simulink model "simulation"  (R2018b)
settings: Solver=ode45  StartTime=0.0  StopTime=inf  MaxStep=0.01  RelTol=1e-3
values from neighbouring files (symbols this model uses):
  A_ref = pi*r^2    (= 0.0188691908756)    [inputsSimulink.m]    (also in stability.m = Geometria(11))
  Cd_lateral1 = Cd_lateral1*A_lateral1/A_ref    (= 119.241996905)    [inputsSimulink.m]
  Cd_lateral2 = Cd_lateral2*A_lateral2/A_ref    (= 238.483993811)    [inputsSimulink.m]
  Cd_paraquedas1 = Cd_paraquedas1*A_paraquedas1/A_ref    (= 24.6433460271)    [inputsSimulink.m]
  Cd_paraquedas2 = Cd_paraquedas2*A_paraquedas2/A_ref    (= 483.857525221)    [inputsSimulink.m]
  Cn = Cn_SB    [inputsSimulink.m]    (also in stability.m = CN_bosters + CN)
  dist_guia = 12    [inputsSimulink.m]
  Empuxo_boster = 4*curvas(:,2)    [inputsSimulink.m]
  g0 = 9.82    [inputsSimulink.m]
  h0 = 1200    [inputsSimulink.m]
  L_coifa = 0.5    [inputsSimulink.m]    (also in stability.m = Geometria(3))
  L_corpo = 2    [inputsSimulink.m]
  Massa_foguete = 1    [inputsSimulink.m]
  Massa_motor_solido = [3.5 1]    [inputsSimulink.m]
  ME = (Cp - CG)/(2*r)    [inputsSimulink.m]
  phi = 0    [inputsSimulink.m]
  r = 0.155/2    (= 0.0775)    [inputsSimulink.m]    (also in stability.m = Geometria(1))
  RE = 6371000    [inputsSimulink.m]
  tempo_abertura1 = 5    [inputsSimulink.m]
  tempo_abertura2 = 7    [inputsSimulink.m]
  tempo_boster = curvas(:,1)    [inputsSimulink.m]
  tempo_motor_solido = [0 tempo_queima_bosters]    [inputsSimulink.m]
  tempo_queima_bosters = max(tempo_boster)    [inputsSimulink.m]
  theta = 0    [inputsSimulink.m]
  Vento_eixo_x = 1    [inputsSimulink.m]
  Vento_eixo_y = 0    [inputsSimulink.m]
libraries: vrlib x3, aerolibatmos2 x1
settings Model: Creator=root  LastModifiedBy=root

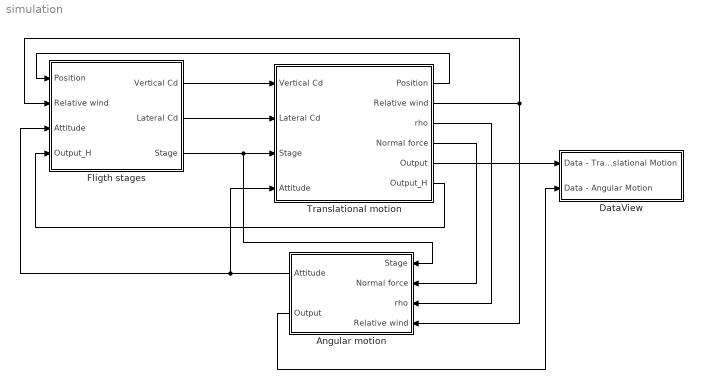
== system simulation ==
  Angular motion : Subsystem
  DataView : Subsystem
  Fligth stages : Subsystem
  Translational motion : Subsystem
  wires:
  Fligth stages/1(Vertical Cd) -> Translational motion/1(Vertical Cd)
  Translational motion/4(Normal force) -> Angular motion/2(Normal force)
  Translational motion/6(Output_H) -> Fligth stages/4(Output_H)
  Translational motion/3(rho) -> Angular motion/3(rho)
  Fligth stages/2(Lateral Cd) -> Translational motion/2(Lateral Cd)
  Fligth stages/3(Stage) -> Angular motion/1(Stage), Translational motion/3(Stage)
  Translational motion/1(Position) -> Fligth stages/1(Position)
  Angular motion/1(Attitude) -> Fligth stages/3(Attitude), Translational motion/4(Attitude)
  Translational motion/2(Relative wind) -> Fligth stages/2(Relative wind), Angular motion/4(Relative wind)
  Translational motion/5(Output) -> DataView/1(Data - Translational Motion)
  Angular motion/2(Output) -> DataView/2(Data - Angular Motion)

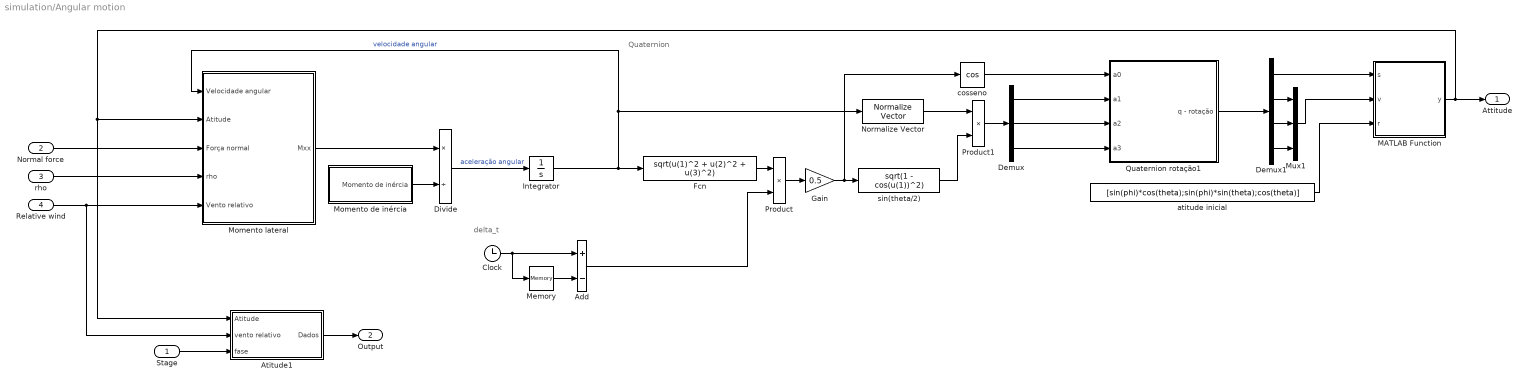
== system simulation/Angular motion ==
  note: Quaternion
  note: delta_t
  Stage : Inport
  Normal force : Inport  Port=2
  rho : Inport  Port=3
  Relative wind : Inport  Port=4
  Add : Sum  Inputs=+-
  Atitude1 : Subsystem
  Clock : Clock
  Demux : Demux  Outputs=3
  Demux1 : Demux
  Divide : Product  Inputs=*/
  Fcn : Fcn  Expr=sqrt(u(1)^2 + u(2)^2 + u(3)^2)
  Gain : Gain  Gain=0.5
  Integrator : Integrator  InitialCondition=[0;0;0]
  MATLAB Function : MATLAB Function  TreatAsAtomicUnit=on
  Memory : Memory
  Momento de inércia : Subsystem
  Momento lateral : Subsystem
  Mux1 : Mux  Inputs=3
  Normalize Vector : vrlib/Utilities/Normalize Vector  maxzero=0
      settings: SourceProductName=Simulink 3D Animation  SourceProductBaseCode=VR
  Product : Product
  Product1 : Product
  Quaternion rotação1 : Subsystem
  atitude inicial : Constant  Value=[sin(phi)*cos(theta);sin(phi)*sin(theta);cos(theta)]
  cosseno : Trigonometry  Operator=cos
  sin(theta/2) : Fcn  Expr=sqrt(1 - cos(u(1))^2)
  Attitude : Outport
  Output : Outport  Port=2
  wires:
  Normal force/1 -> Momento lateral/3(Força normal)
  rho/1 -> Momento lateral/4(rho)
  Relative wind/1 -> Momento lateral/5(Vento relativo), Atitude1/2(vento relativo)
  Momento lateral/1(Mxx) -> Divide/1
  Momento de inércia/1(Momento de inércia) -> Divide/2
  Divide/1 -> Integrator/1  "aceleração angular"
  Clock/1 -> Memory/1, Add/1
  Memory/1 -> Add/2
  Integrator/1 -> Normalize Vector/1, Momento lateral/1(Velocidade angular), Fcn/1  "velocidade angular"
  Add/1 -> Product/2
  Product/1 -> Gain/1
  Gain/1 -> cosseno/1, sin(theta/2)/1
  sin(theta/2)/1 -> Product1/2
  Product1/1 -> Demux/1
  cosseno/1 -> Quaternion rotação1/1(a0)
  atitude inicial/1 -> MATLAB Function/3(r)
  MATLAB Function/1(y) -> Atitude1/1(Atitude), Momento lateral/2(Atitude), Attitude/1
  Fcn/1 -> Product/1
  Normalize Vector/1 -> Product1/1
  Demux/3 -> Quaternion rotação1/4(a3)
  Demux/2 -> Quaternion rotação1/3(a2)
  Demux/1 -> Quaternion rotação1/2(a1)
  Demux1/1 -> MATLAB Function/1(s)
  Demux1/4 -> Mux1/3
  Demux1/3 -> Mux1/2
  Demux1/2 -> Mux1/1
  Mux1/1 -> MATLAB Function/2(v)
  Quaternion rotação1/1(q - rotação) -> Demux1/1
  Stage/1 -> Atitude1/3(fase)
  Atitude1/1(Dados) -> Output/1

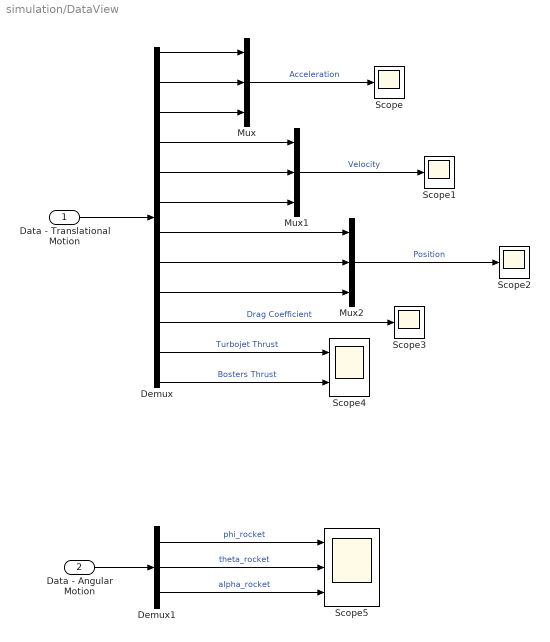
== system simulation/DataView ==
  Data - Translational Motion : Inport
  Data - Angular Motion : Inport  Port=2
  Demux : Demux  Outputs=12
  Demux1 : Demux  Outputs=3
  Mux : Mux  Inputs=3
  Mux1 : Mux  Inputs=3
  Mux2 : Mux  Inputs=3
  Scope{,1..3} (4 alike) : Scope
  Scope4 : Scope  NumInputPorts=2
  Scope5 : Scope  NumInputPorts=3
  wires:
  Data - Translational Motion/1 -> Demux/1
  Demux/1 -> Mux/1
  Demux/2 -> Mux/2
  Demux/3 -> Mux/3
  Demux/4 -> Mux1/1
  Demux/5 -> Mux1/2
  Demux/6 -> Mux1/3
  Demux/7 -> Mux2/1
  Demux/8 -> Mux2/2
  Demux/9 -> Mux2/3
  Mux/1 -> Scope/1  "Acceleration"
  Mux1/1 -> Scope1/1  "Velocity"
  Mux2/1 -> Scope2/1  "Position"
  Demux/10 -> Scope3/1  "Drag Coefficient"
  Demux/11 -> Scope4/1  "Turbojet Thrust"
  Demux/12 -> Scope4/2  "Bosters Thrust"
  Data - Angular Motion/1 -> Demux1/1
  Demux1/2 -> Scope5/2  "theta_rocket"
  Demux1/3 -> Scope5/3  "alpha_rocket"
  Demux1/1 -> Scope5/1  "phi_rocket"

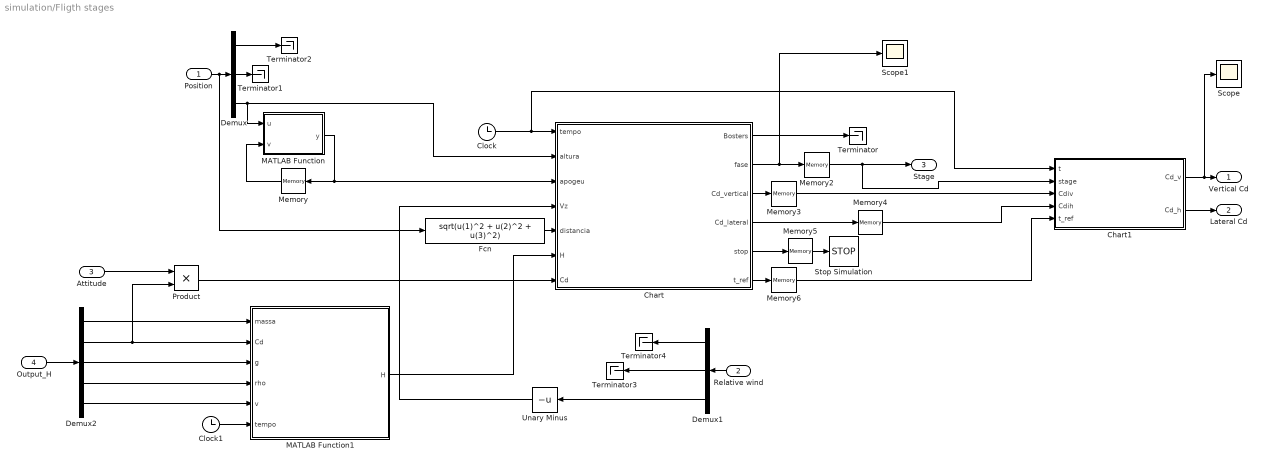
== system simulation/Fligth stages ==
  Position : Inport
  Relative wind : Inport  Port=2
  Attitude : Inport  Port=3
  Output_H : Inport  Port=4
  Chart : Stateflow chart  TreatAsAtomicUnit=on
  Chart1 : Stateflow chart  TreatAsAtomicUnit=on
  Clock : Clock
  Clock1 : Clock
  Demux : Demux  Outputs=3
  Demux1 : Demux  Outputs=3
  Demux2 : Demux  Outputs=5
  Fcn : Fcn  Expr=sqrt(u(1)^2 + u(2)^2 + u(3)^2)
  MATLAB Function : MATLAB Function  TreatAsAtomicUnit=on
  MATLAB Function1 : MATLAB Function  TreatAsAtomicUnit=on
  Memory{,2..6} (6 alike) : Memory
  Product : Product
  Scope : Scope
  Scope1 : Scope
  Stop Simulation : Stop
  Terminator{,1..4} (5 alike) : Terminator
  Unary Minus : UnaryMinus
  Vertical Cd : Outport
  Lateral Cd : Outport  Port=2
  Stage : Outport  Port=3
  wires:
  Demux/3 -> MATLAB Function/1(u), Chart/2(altura)
  Chart/2(fase) -> Scope1/1, Memory2/1
  Chart/3(Cd_vertical) -> Memory3/1
  Chart/4(Cd_lateral) -> Memory4/1
  Position/1 -> Fcn/1, Demux/1
  Demux/2 -> Terminator1/1
  Demux/1 -> Terminator2/1
  Chart/5(stop) -> Memory5/1
  Relative wind/1 -> Demux1/1
  Demux1/2 -> Terminator3/1
  Demux1/1 -> Terminator4/1
  Demux1/3 -> Unary Minus/1
  Unary Minus/1 -> Chart/4(Vz)
  Fcn/1 -> Chart/5(distancia)
  MATLAB Function/1(y) -> Chart/3(apogeu), Memory/1
  Memory/1 -> MATLAB Function/2(v)
  Output_H/1 -> Demux2/1
  Demux2/1 -> MATLAB Function1/1(massa)
  Demux2/2 -> Product/2, MATLAB Function1/2(Cd)
  Demux2/3 -> MATLAB Function1/3(g)
  Demux2/4 -> MATLAB Function1/4(rho)
  Demux2/5 -> MATLAB Function1/5(v)
  MATLAB Function1/1(H) -> Chart/6(H)
  Clock/1 -> Chart1/1(t), Chart/1(tempo)
  Chart/6(t_ref) -> Memory6/1
  Chart1/2(Cd_h) -> Lateral Cd/1
  Attitude/1 -> Product/1
  Product/1 -> Chart/7(Cd)
  Clock1/1 -> MATLAB Function1/6(tempo)
  Memory2/1 -> Stage/1, Chart1/2(stage)
  Memory3/1 -> Chart1/3(Cdiv)
  Memory4/1 -> Chart1/4(Cdih)
  Memory5/1 -> Stop Simulation/1
  Memory6/1 -> Chart1/5(t_ref)
  Chart1/1(Cd_v) -> Scope/1, Vertical Cd/1
  Chart/1(Bosters) -> Terminator/1

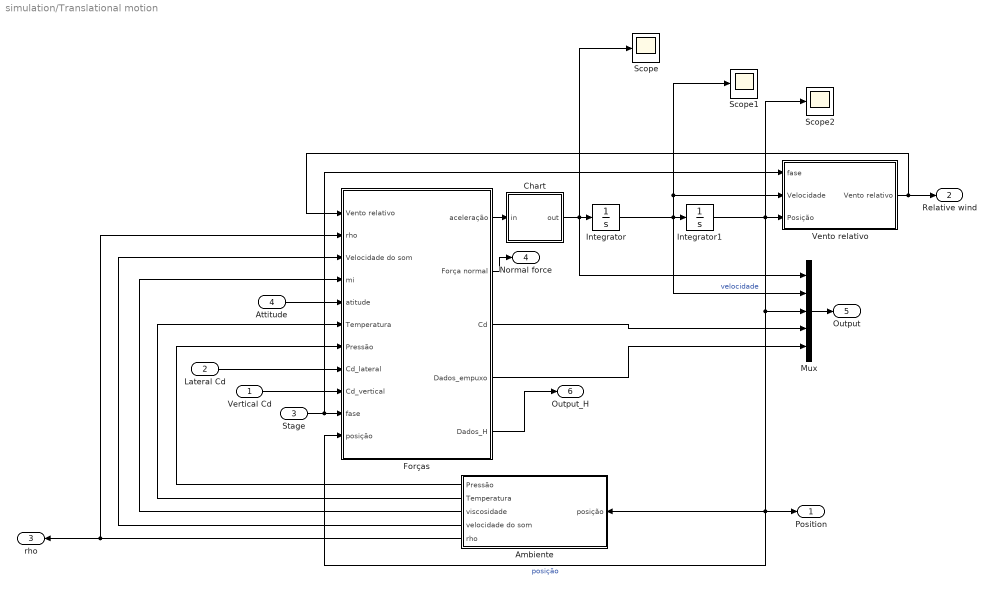
== system simulation/Translational motion ==
  Vertical Cd : Inport
  Lateral Cd : Inport  Port=2
  Stage : Inport  Port=3
  Attitude : Inport  Port=4
  Ambiente : Subsystem
  Chart : Stateflow chart  TreatAsAtomicUnit=on
  Forças : Subsystem
  Integrator : Integrator  InitialCondition=[0;0;0]
  Integrator1 : Integrator  InitialCondition=[0; 0; 0]
  Mux : Mux  Inputs=5
  Scope : Scope
  Scope1 : Scope
  Scope2 : Scope
  Vento relativo : Subsystem
  Position : Outport
  Relative wind : Outport  Port=2
  rho : Outport  Port=3
  Normal force : Outport  Port=4
  Output : Outport  Port=5
  Output_H : Outport  Port=6
  wires:
  Integrator/1 -> Scope1/1, Vento relativo/2(Velocidade), Mux/2, Integrator1/1  "velocidade"
  Integrator1/1 -> Scope2/1, Vento relativo/3(Posição), Position/1, Forças/11(posição), Ambiente/1(posição), Mux/3  "posição"
  Attitude/1 -> Forças/5(atitude)
  Vento relativo/1(Vento relativo) -> Relative wind/1, Forças/1(Vento relativo)
  Ambiente/5(rho) -> Forças/2(rho), rho/1
  Ambiente/4(velocidade do som) -> Forças/3(Velocidade do som)
  Ambiente/3(viscosidade) -> Forças/4(mi)
  Ambiente/2(Temperatura) -> Forças/6(Temperatura)
  Ambiente/1(Pressão) -> Forças/7(Pressão)
  Forças/2(Força normal) -> Normal force/1
  Lateral Cd/1 -> Forças/8(Cd_lateral)
  Vertical Cd/1 -> Forças/9(Cd_vertical)
  Forças/1(aceleração) -> Chart/1(in)
  Chart/1(out) -> Scope/1, Mux/1, Integrator/1
  Stage/1 -> Vento relativo/1(fase), Forças/10(fase)
  Mux/1 -> Output/1
  Forças/3(Cd) -> Mux/4
  Forças/4(Dados_empuxo) -> Mux/5
  Forças/5(Dados_H) -> Output_H/1

== system simulation/Angular motion/Atitude1 ==
  Atitude : Inport
  vento relativo : Inport  Port=2
  fase : Inport  Port=3
  Chart : Stateflow chart  TreatAsAtomicUnit=on
  Demux : Demux  Outputs=3
  MATLAB Function : MATLAB Function  TreatAsAtomicUnit=on
  Mux : Mux  Inputs=3
  Dados : Outport
  wires:
  Atitude/1 -> MATLAB Function/3(a), Demux/1
  Demux/1 -> Chart/1(Px)
  Demux/2 -> Chart/2(Py)
  Demux/3 -> Chart/3(Pz)
  vento relativo/1 -> MATLAB Function/2(v)
  fase/1 -> Chart/4(fase), MATLAB Function/1(fase)
  Chart/1(phi) -> Mux/1
  Chart/2(theta) -> Mux/2
  MATLAB Function/1(alfa) -> Mux/3
  Mux/1 -> Dados/1

== system simulation/Angular motion/Momento de inércia ==
  Constant : Constant
  Momento de inércia : Outport
  wires:
  Constant/1 -> Momento de inércia/1

== system simulation/Angular motion/Momento lateral ==
  Velocidade angular : Inport
  Atitude : Inport  Port=2
  Força normal : Inport  Port=3
  rho : Inport  Port=4
  Vento relativo : Inport  Port=5
  Lateral torque : Subsystem
  Mxx : Outport
  wires:
  Velocidade angular/1 -> Lateral torque/1(Velocidade angular)
  Atitude/1 -> Lateral torque/2(Atitude)
  Força normal/1 -> Lateral torque/3(Força normal)
  rho/1 -> Lateral torque/4(rho)
  Vento relativo/1 -> Lateral torque/5(Vento relativo)
  Lateral torque/1(Mxx) -> Mxx/1

== system simulation/Angular motion/Quaternion rotação1 ==
  a0 : Inport
  a1 : Inport  Port=2
  a2 : Inport  Port=3
  a3 : Inport  Port=4
  Chart : Stateflow chart  TreatAsAtomicUnit=on
  Clock1 : Clock
  Memory : Memory  InitialCondition=[0 0 0 0]
  q - rotação : Outport
  wires:
  Clock1/1 -> Chart/1(time)
  Chart/2(d) -> Memory/1
  Chart/1(y) -> q - rotação/1
  Memory/1 -> Chart/6(c)
  a0/1 -> Chart/2(a0)
  a1/1 -> Chart/3(a1)
  a2/1 -> Chart/4(a2)
  a3/1 -> Chart/5(a3)

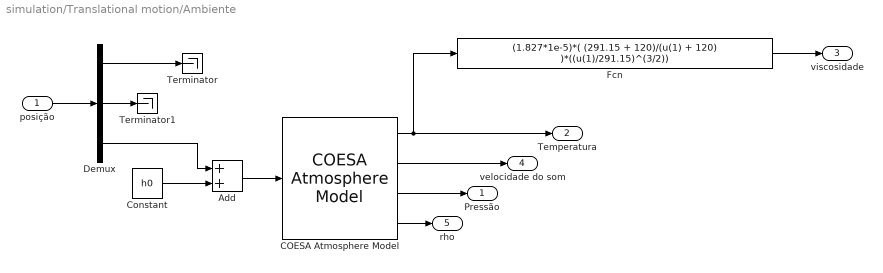
== system simulation/Translational motion/Ambiente ==
  posição : Inport
  Add : Sum
  COESA Atmosphere Model : aerolibatmos2/COESA Atmosphere Model  units=Metric (MKS)  spec=1976 COESA-extended U.S. Standard Atmosphere  model=Profile  profile_var=High temperature  profile_percent=1%  profile_alt=5 km (16404 ft)  envelope_var=High temperature  envelope_percent=1%  action=Warning
  Constant : Constant  Value=h0
  Demux : Demux  Outputs=3
  Fcn : Fcn  Expr=(1.827*1e-5)*( (291.15 + 120)/(u(1) + 120) )*((u(1)/291.15)^(3/2))
  Terminator : Terminator
  Terminator1 : Terminator
  Pressão : Outport
  Temperatura : Outport  Port=2
  viscosidade : Outport  Port=3
  velocidade do som : Outport  Port=4
  rho : Outport  Port=5
  wires:
  COESA Atmosphere Model/1 -> Fcn/1, Temperatura/1
  COESA Atmosphere Model/2 -> velocidade do som/1
  COESA Atmosphere Model/3 -> Pressão/1
  COESA Atmosphere Model/4 -> rho/1
  posição/1 -> Demux/1
  Demux/1 -> Terminator/1
  Demux/2 -> Terminator1/1
  Demux/3 -> Add/1
  Fcn/1 -> viscosidade/1
  Add/1 -> COESA Atmosphere Model/1
  Constant/1 -> Add/2

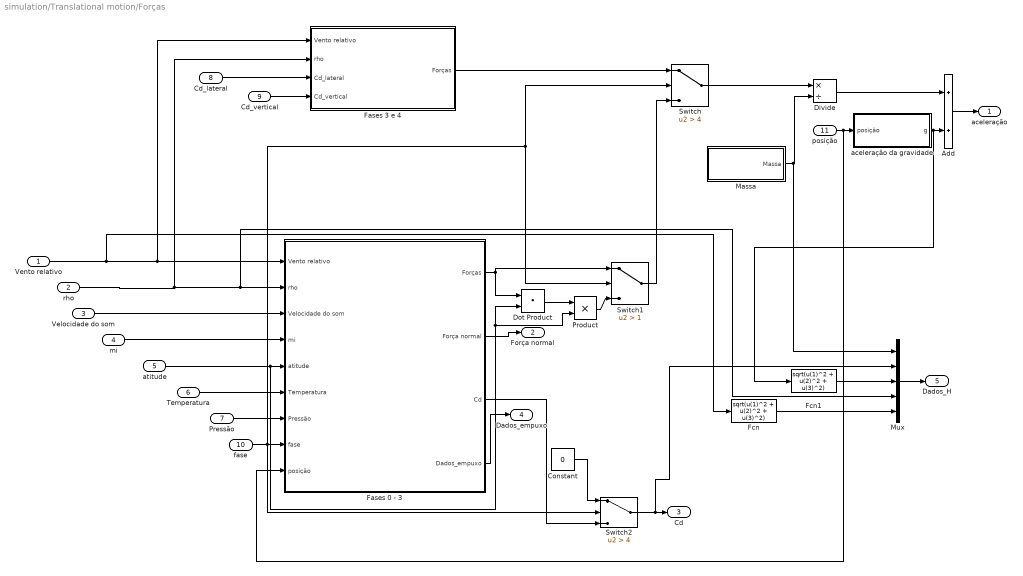
== system simulation/Translational motion/Forças ==
  Vento relativo : Inport
  rho : Inport  Port=2
  Velocidade do som : Inport  Port=3
  mi : Inport  Port=4
  atitude : Inport  Port=5
  Temperatura : Inport  Port=6
  Pressão : Inport  Port=7
  Cd_lateral : Inport  Port=8
  Cd_vertical : Inport  Port=9
  fase : Inport  Port=10
  posição : Inport  Port=11
  Add : Sum
  Constant : Constant  Value=0
  Divide : Product  Inputs=*/
  Dot Product : DotProduct  InputSameDT=on  OutDataTypeStr=Inherit: Inherit via internal rule
  Fases 0 - 3 : Subsystem
  Fases 3 e 4 : Subsystem
  Fcn : Fcn  Expr=sqrt(u(1)^2 + u(2)^2 + u(3)^2)
  Fcn1 : Fcn  Expr=sqrt(u(1)^2 + u(2)^2 + u(3)^2)
  Massa : Subsystem
  Mux : Mux  Inputs=5
  Product : Product
  Switch : Switch  Criteria=u2 > Threshold  Threshold=4
  Switch1 : Switch  Criteria=u2 > Threshold  Threshold=1
  Switch2 : Switch  Criteria=u2 > Threshold  Threshold=4
  aceleração da gravidade : Subsystem
  aceleração : Outport
  Força normal : Outport  Port=2
  Cd : Outport  Port=3
  Dados_empuxo : Outport  Port=4
  Dados_H : Outport  Port=5
  wires:
  Add/1 -> aceleração/1
  aceleração da gravidade/1(g) -> Fcn1/1, Add/2
  rho/1 -> Fases 3 e 4/2(rho), Mux/4, Fases 0 - 3/2(rho)
  Velocidade do som/1 -> Fases 0 - 3/3(Velocidade do som)
  mi/1 -> Fases 0 - 3/4(mi)
  Temperatura/1 -> Fases 0 - 3/6(Temperatura)
  Pressão/1 -> Fases 0 - 3/7(Pressão)
  Fases 0 - 3/2(Força normal) -> Força normal/1
  Switch1/1 -> Switch/3
  Fases 3 e 4/1(Forças) -> Switch/1
  Cd_lateral/1 -> Fases 3 e 4/3(Cd_lateral)
  Cd_vertical/1 -> Fases 3 e 4/4(Cd_vertical)
  Switch/1 -> Divide/1
  Massa/1(Massa) -> Mux/1, Divide/2
  Divide/1 -> Add/1
  Fases 0 - 3/1(Forças) -> Switch1/1, Dot Product/1
  atitude/1 -> Product/2, Dot Product/2, Fases 0 - 3/5(atitude)
  Dot Product/1 -> Product/1
  Product/1 -> Switch1/3
  Switch2/1 -> Mux/2, Cd/1
  Constant/1 -> Switch2/1
  Fases 0 - 3/3(Cd) -> Switch2/3
  Fases 0 - 3/4(Dados_empuxo) -> Dados_empuxo/1
  fase/1 -> Switch2/2, Switch/2, Switch1/2, Fases 0 - 3/8(fase)
  posição/1 -> Fases 0 - 3/9(posição), aceleração da gravidade/1(posição)
  Mux/1 -> Dados_H/1
  Vento relativo/1 -> Fcn/1, Fases 3 e 4/1("Vento relativo "), Fases 0 - 3/1(Vento relativo)
  Fcn/1 -> Mux/5
  Fcn1/1 -> Mux/3

== system simulation/Translational motion/Vento relativo ==
  fase : Inport
  Velocidade : Inport  Port=2
  Posição : Inport  Port=3
  Add : Sum
  Add1 : Sum
  Clock : Clock
  Demux : Demux  Outputs=3
  Mux : Mux  Inputs=3
  Scope : Scope  NumInputPorts=2
  Unary Minus : UnaryMinus
  Vento : MATLAB Function  TreatAsAtomicUnit=on
  Vento relativo : Outport
  wires:
  Velocidade/1 -> Unary Minus/1
  Demux/1 -> Add/2
  Add/1 -> Mux/1
  Demux/2 -> Add1/2
  Add1/1 -> Mux/2
  Demux/3 -> Mux/3
  Unary Minus/1 -> Demux/1
  Posição/1 -> Vento/2(posicao)
  Clock/1 -> Vento/3(tempo)
  Vento/1(vento_x) -> Add/1, Scope/1
  Vento/2(vento_y) -> Add1/1, Scope/2
  Mux/1 -> Vento relativo/1
  fase/1 -> Vento/1(fase)

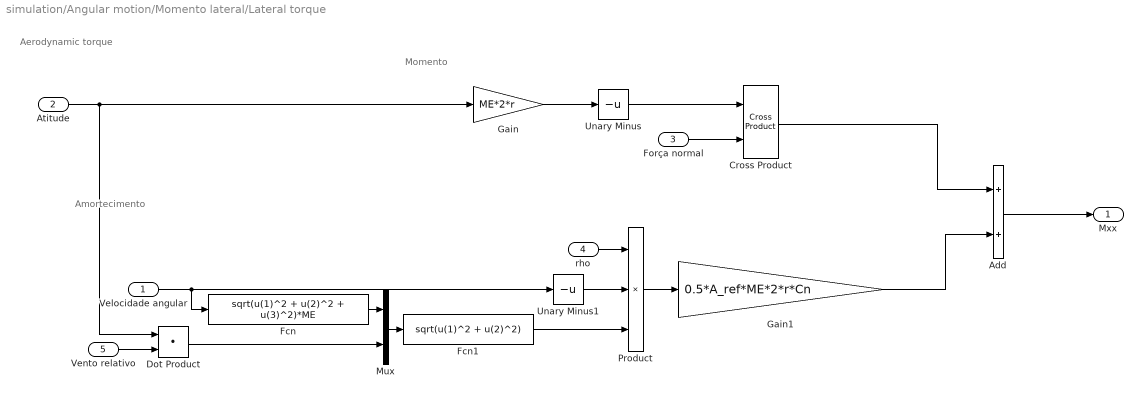
== system simulation/Angular motion/Momento lateral/Lateral torque ==
  note: Amortecimento
  note: Momento
  note: Aerodynamic torque
  Velocidade angular : Inport
  Atitude : Inport  Port=2
  Força normal : Inport  Port=3
  rho : Inport  Port=4
  Vento relativo : Inport  Port=5
  Add : Sum
  Cross Product : vrlib/Utilities/Cross Product
      settings: SourceProductBaseCode=VR
  Dot Product : DotProduct  InputSameDT=on  OutDataTypeStr=Inherit: Inherit via internal rule
  Fcn : Fcn  Expr=sqrt(u(1)^2 + u(2)^2 + u(3)^2)*ME
  Fcn1 : Fcn  Expr=sqrt(u(1)^2 + u(2)^2)
  Gain : Gain  Gain=ME*2*r
  Gain1 : Gain  Gain=0.5*A_ref*ME*2*r*Cn
  Mux : Mux  Inputs=2
  Product : Product  Inputs=3
  Unary Minus : UnaryMinus
  Unary Minus1 : UnaryMinus
  Mxx : Outport
  wires:
  Cross Product/1 -> Add/1
  Unary Minus/1 -> Cross Product/1
  Product/1 -> Gain1/1
  Gain1/1 -> Add/2
  Gain/1 -> Unary Minus/1
  Unary Minus1/1 -> Product/2
  Força normal/1 -> Cross Product/2
  rho/1 -> Product/1
  Atitude/1 -> Dot Product/1, Gain/1
  Velocidade angular/1 -> Fcn/1, Unary Minus1/1
  Fcn/1 -> Mux/1
  Mux/1 -> Fcn1/1
  Fcn1/1 -> Product/3
  Dot Product/1 -> Mux/2
  Vento relativo/1 -> Dot Product/2
  Add/1 -> Mxx/1

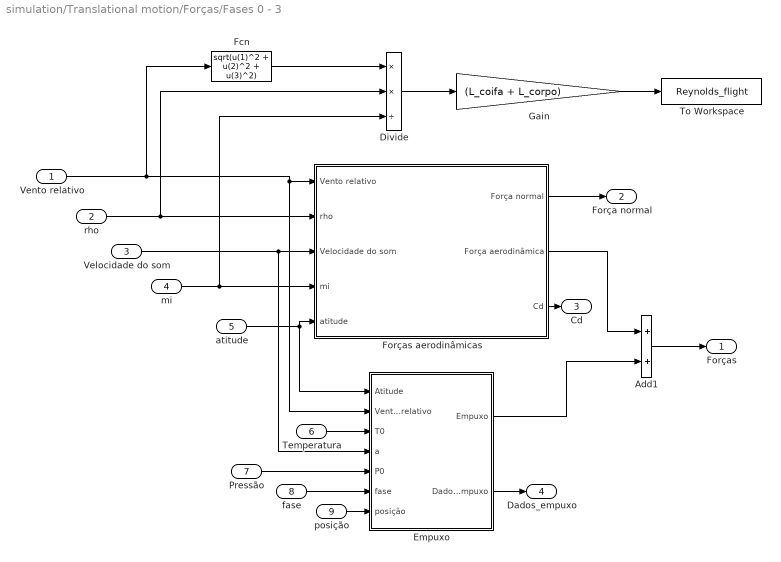
== system simulation/Translational motion/Forças/Fases 0 - 3 ==
  Vento relativo : Inport
  rho : Inport  Port=2
  Velocidade do som : Inport  Port=3
  mi : Inport  Port=4
  atitude : Inport  Port=5
  Temperatura : Inport  Port=6
  Pressão : Inport  Port=7
  fase : Inport  Port=8
  posição : Inport  Port=9
  Add1 : Sum
  Divide : Product  Inputs=**/
  Empuxo : Subsystem
  Fcn : Fcn  Expr=sqrt(u(1)^2 + u(2)^2 + u(3)^2)
  Forças aerodinâmicas : Subsystem
  Gain : Gain  Gain=(L_coifa + L_corpo)
  To Workspace : ToWorkspace  VariableName=Reynolds_flight  SaveFormat=Timeseries  SampleTime=-1
  Forças : Outport
  Força normal : Outport  Port=2
  Cd : Outport  Port=3
  Dados_empuxo : Outport  Port=4
  wires:
  Forças aerodinâmicas/1(Força normal) -> Força normal/1
  Empuxo/1(Empuxo) -> Add1/2
  rho/1 -> Divide/2, Forças aerodinâmicas/2(rho)
  Vento relativo/1 -> Fcn/1, Forças aerodinâmicas/1(Vento relativo), Empuxo/2(Vento relativo)
  Add1/1 -> Forças/1
  Forças aerodinâmicas/2(Força aerodinâmica) -> Add1/1
  Velocidade do som/1 -> Empuxo/4(a), Forças aerodinâmicas/3(Velocidade do som)
  atitude/1 -> Empuxo/1(Atitude), Forças aerodinâmicas/5(atitude)
  Pressão/1 -> Empuxo/5(P0)
  mi/1 -> Divide/3, Forças aerodinâmicas/4(mi)
  Temperatura/1 -> Empuxo/3(T0)
  fase/1 -> Empuxo/6(fase)
  Forças aerodinâmicas/3(Cd) -> Cd/1
  Empuxo/2(Dados_empuxo) -> Dados_empuxo/1
  posição/1 -> Empuxo/7(posição)
  Divide/1 -> Gain/1
  Gain/1 -> To Workspace/1
  Fcn/1 -> Divide/1

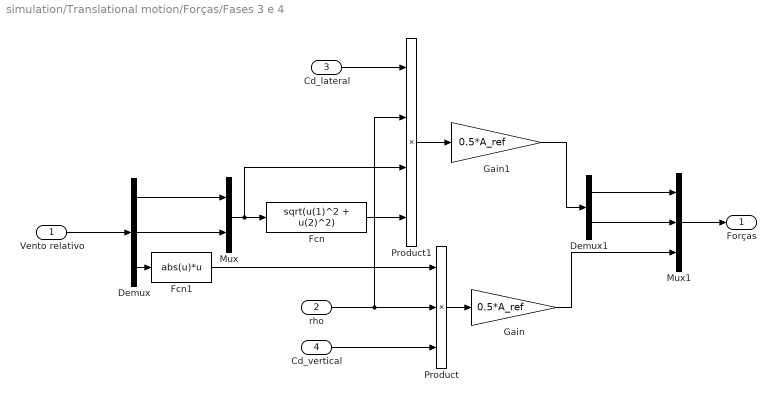
== system simulation/Translational motion/Forças/Fases 3 e 4 ==
  "Vento relativo " : Inport
  rho : Inport  Port=2
  Cd_lateral : Inport  Port=3
  Cd_vertical : Inport  Port=4
  Demux : Demux  Outputs=3
  Demux1 : Demux  Outputs=2
  Fcn : Fcn  Expr=sqrt(u(1)^2 + u(2)^2)
  Fcn1 : Fcn  Expr=abs(u)*u
  Gain : Gain  Gain=0.5*A_ref
  Gain1 : Gain  Gain=0.5*A_ref
  Mux : Mux  Inputs=2
  Mux1 : Mux  Inputs=3
  Product : Product  Inputs=3
  Product1 : Product  Inputs=4
  Forças : Outport
  wires:
  "Vento relativo "/1 -> Demux/1
  Demux/1 -> Mux/1
  Demux/2 -> Mux/2
  Demux/3 -> Fcn1/1
  rho/1 -> Product1/2, Product/2
  Cd_vertical/1 -> Product/3
  Fcn1/1 -> Product/1
  Product/1 -> Gain/1
  Fcn/1 -> Product1/4
  Mux/1 -> Product1/3, Fcn/1
  Cd_lateral/1 -> Product1/1
  Product1/1 -> Gain1/1
  Gain1/1 -> Demux1/1
  Gain/1 -> Mux1/3
  Mux1/1 -> Forças/1
  Demux1/2 -> Mux1/2
  Demux1/1 -> Mux1/1

== system simulation/Translational motion/Forças/Massa ==
  1-D Lookup Table : Lookup_n-D  NumberOfTableDimensions=1  BreakpointsForDimension1=tempo_motor_solido  Table=Massa_motor_solido  InternalRulePriority=Speed  RndMeth=Simplest  InputSameDT=on
  Add : Sum
  Clock : Clock
  Constant : Constant  Value=Massa_foguete
  Constant1 : Constant  Value=Massa_motor_solido(2)
  Scope : Scope
  Switch : Switch  Criteria=u2 > Threshold  Threshold=tempo_queima_bosters
  Massa : Outport
  wires:
  Add/1 -> Massa/1, Scope/1
  Constant/1 -> Add/1
  Switch/1 -> Add/2
  Clock/1 -> Switch/2, 1-D Lookup Table/1
  1-D Lookup Table/1 -> Switch/3
  Constant1/1 -> Switch/1

== system simulation/Translational motion/Forças/aceleração da gravidade ==
  posição : Inport
  Constant : Constant  Value=0
  Demux : Demux  Outputs=3
  Fcn : Fcn  Expr=-g0*(RE^2)/((RE + u(1))^2)
  Mux : Mux  Inputs=3
  Scope : Scope  NumInputPorts=2
  Terminator : Terminator
  Terminator1 : Terminator
  g : Outport
  wires:
  posição/1 -> Demux/1
  Demux/1 -> Terminator/1
  Demux/2 -> Terminator1/1
  Demux/3 -> Scope/2, Fcn/1
  Fcn/1 -> Scope/1, Mux/3  "g"
  Mux/1 -> g/1
  Constant/1 -> Mux/2, Mux/1

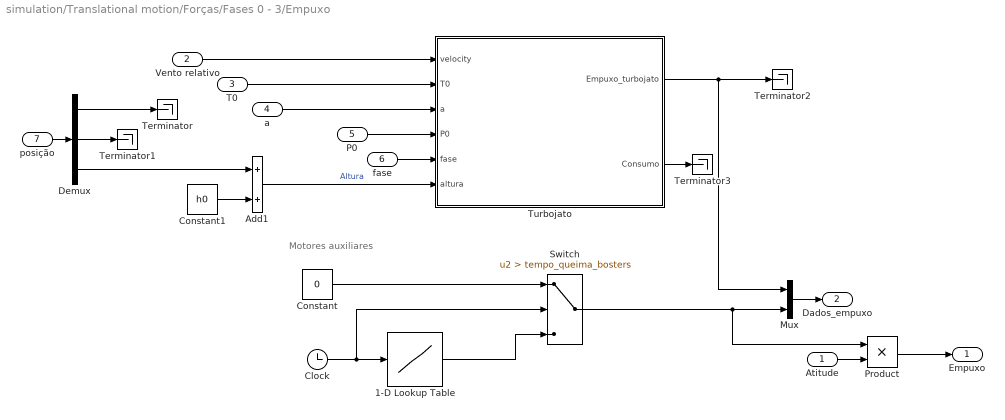
== system simulation/Translational motion/Forças/Fases 0 - 3/Empuxo ==
  note: Motores auxiliares
  Atitude : Inport
  Vento relativo : Inport  Port=2
  T0 : Inport  Port=3
  a : Inport  Port=4
  P0 : Inport  Port=5
  fase : Inport  Port=6
  posição : Inport  Port=7
  1-D Lookup Table : Lookup_n-D  NumberOfTableDimensions=1  BreakpointsForDimension1=tempo_boster  Table=Empuxo_boster  InternalRulePriority=Speed  RndMeth=Simplest  InputSameDT=on
  Add1 : Sum
  Clock : Clock
  Constant : Constant  Value=0
  Constant1 : Constant  Value=h0
  Demux : Demux  Outputs=3
  Mux : Mux  Inputs=2
  Product : Product
  Switch : Switch  Criteria=u2 > Threshold  Threshold=tempo_queima_bosters
  Terminator{,1..3} (4 alike) : Terminator
  Turbojato : MATLAB Function  TreatAsAtomicUnit=on
  Empuxo : Outport
  Dados_empuxo : Outport  Port=2
  wires:
  Vento relativo/1 -> Turbojato/1(velocity)
  T0/1 -> Turbojato/2(T0)
  P0/1 -> Turbojato/4(P0)
  a/1 -> Turbojato/3(a)
  Clock/1 -> 1-D Lookup Table/1, Switch/2
  1-D Lookup Table/1 -> Switch/3
  Constant/1 -> Switch/1
  Switch/1 -> Product/1, Mux/2
  Atitude/1 -> Product/2
  Product/1 -> Empuxo/1
  Mux/1 -> Dados_empuxo/1
  Turbojato/2(Consumo) -> Terminator3/1
  posição/1 -> Demux/1
  Demux/3 -> Add1/1
  Demux/1 -> Terminator/1
  Demux/2 -> Terminator1/1
  Add1/1 -> Turbojato/6(altura)  "Altura"
  Constant1/1 -> Add1/2
  Turbojato/1(Empuxo_turbojato) -> Mux/1, Terminator2/1
  fase/1 -> Turbojato/5(fase)

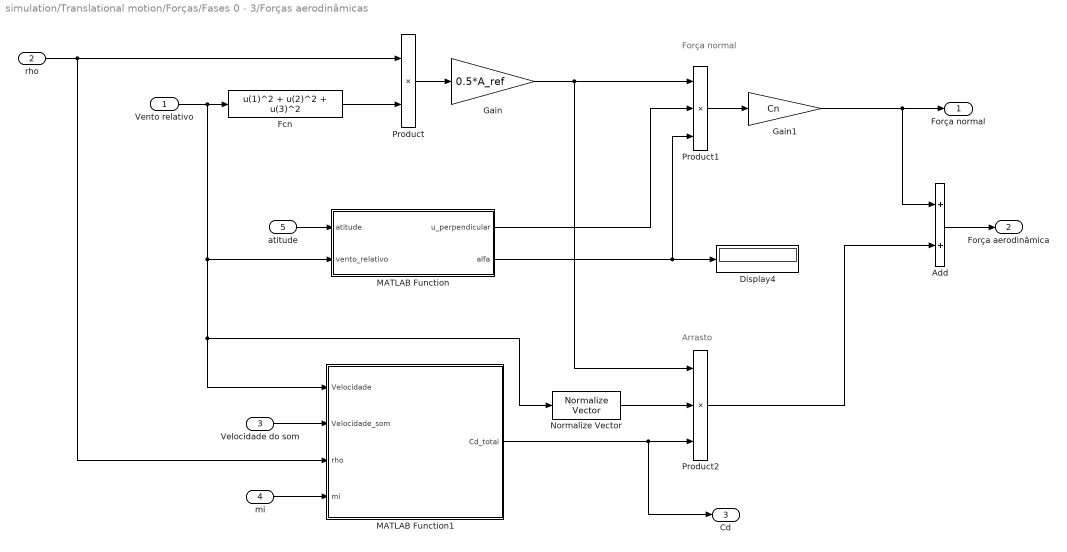
== system simulation/Translational motion/Forças/Fases 0 - 3/Forças aerodinâmicas ==
  note: Arrasto
  note: Força normal
  Vento relativo : Inport
  rho : Inport  Port=2
  Velocidade do som : Inport  Port=3
  mi : Inport  Port=4
  atitude : Inport  Port=5
  Add : Sum
  Display4 : Display
  Fcn : Fcn  Expr=u(1)^2 + u(2)^2 + u(3)^2
  Gain : Gain  Gain=0.5*A_ref
  Gain1 : Gain  Gain=Cn
  MATLAB Function : MATLAB Function  TreatAsAtomicUnit=on
  MATLAB Function1 : MATLAB Function  TreatAsAtomicUnit=on
  Normalize Vector : vrlib/Utilities/Normalize Vector  maxzero=0
      settings: SourceProductName=Simulink 3D Animation  SourceProductBaseCode=VR
  Product : Product
  Product1 : Product  Inputs=3
  Product2 : Product  Inputs=3
  Força normal : Outport
  Força aerodinâmica : Outport  Port=2
  Cd : Outport  Port=3
  wires:
  Fcn/1 -> Product/2
  rho/1 -> MATLAB Function1/3(rho), Product/1
  Product/1 -> Gain/1
  Gain/1 -> Product2/1, Product1/1
  MATLAB Function/1(u_perpendicular) -> Product1/2
  MATLAB Function/2(alfa) -> Display4/1, Product1/3
  Product1/1 -> Gain1/1
  MATLAB Function1/1(Cd_total) -> Cd/1, Product2/3
  Gain1/1 -> Força normal/1, Add/1
  Product2/1 -> Add/2
  Add/1 -> Força aerodinâmica/1
  Velocidade do som/1 -> MATLAB Function1/2(Velocidade_som)
  mi/1 -> MATLAB Function1/4(mi)
  Normalize Vector/1 -> Product2/2
  atitude/1 -> MATLAB Function/1(atitude)
  Vento relativo/1 -> MATLAB Function1/1(Velocidade), Normalize Vector/1, MATLAB Function/2(vento_relativo), Fcn/1

== stateflow chart simulation/Fligth stages/Chart1 ==
  state State1
    during:
    Cd_v = Cdiv + (t - t_ref) * (Cd_paraquedas1 - Cdiv) / tempo_abertura1;
    Cd_h = Cdih + (t - t_ref) * (Cd_lateral1 - Cdih) / tempo_abertura1;
  state State2
    entry:
    Cd_v = Cd_paraquedas1;
    Cd_h = Cd_lateral1;
  state State0
    entry:
    Cd_v = 0;
    Cd_h = 0;
  state State3
    during:
    Cd_v = Cdiv + (t - t_ref) * (Cd_paraquedas2 - Cdiv) / tempo_abertura2;
    Cd_h = Cdih + (t - t_ref) * (Cd_lateral2 - Cdih) / tempo_abertura2;
  state State4
    entry:
    Cd_v = Cd_paraquedas2;
    Cd_h = Cd_lateral2;
  State0 -> State1 : [stage >= 5]
  State1 -> State2 : [(t - t_ref) >= tempo_abertura1]
  State2 -> State3 : [stage >= 6]
  (default) -> State0
  State3 -> State4 : [(t - t_ref) >= tempo_abertura2]
  data: t input; tempo_abertura1 parameter; Cd_lateral1 parameter; Cd_paraquedas2 parameter; tempo_abertura2 parameter; Cd_lateral2 parameter; Cd_paraquedas1 parameter; stage input; Cdiv input; Cdih input; t_ref input; Cd_v output; Cd_h output

== stateflow chart simulation/Fligth stages/Chart ==
  state State1
    entry:
    fase = 1;
    Bosters = 0;
    Cd_vertical = 0;
    Cd_lateral = 0;
    stop = 0;
    t_ref = tempo;
  state State5
    entry:
    fase = 5;
    Bosters = 0;
    Cd_vertical = Cd(3);
    Cd_lateral = sqrt(Cd(1)^2 + Cd(2)^2);
    stop = 0;
    t_ref = tempo;
  state State6
    entry:
    fase = 6;
    Bosters = 0;
    Cd_vertical = Cd_paraquedas1;
    Cd_lateral = Cd_lateral1;
    stop = 0;
    t_ref = tempo;
  state State0
    entry:
    fase = 0;
    Bosters = 1;
    Cd_vertical = 0;
    Cd_lateral = 0;
    stop = 0;
    t_ref = tempo;
  state State3
    entry:
    fase = 3;
    Bosters = 0;
    Cd_vertical = 0;
    Cd_lateral = 0;
    stop = 0;
    t_ref = tempo;
  state State2
    entry:
    fase = 2;
    Bosters = 1;
    Cd_vertical = 0;
    Cd_lateral = 0;
    stop = 0;
    t_ref = tempo;
  state State7
    entry:
    fase = 7;
    Bosters = 0;
    Cd_vertical = Cd_paraquedas2;
    Cd_lateral = Cd_lateral2;
    stop = 1;
    t_ref = tempo;
  State0 -> State1 [order 1] : [(tempo > tempo_queima_bosters) && (distancia < dist_guia)]
  State5 -> State6 [order 1] : [altura < 0.2*apogeu]
  State1 -> State3 : [distancia > dist_guia]
  (default) -> State0
  State3 -> State5 [order 2] : [(altura < 0.99*apogeu) && (Vz < 0)]
  State5 -> State7 [order 2] : [altura <=0]
  State6 -> State7 : [altura <= 0]
  State2 -> State3 [order 1] : [tempo > tempo_queima_bosters]
  State3 -> State7 [order 1] : [altura <=0]
  State0 -> State2 [order 2] : [(tempo < tempo_queima_bosters) && (distancia > dist_guia)]
  State2 -> State7 [order 2] : [altura <= 0]
  data: tempo input; altura input; apogeu input; Cd_paraquedas1 parameter; Cd_lateral1 parameter; Cd_lateral2 parameter; Cd_paraquedas2 parameter; tempo_queima_bosters parameter; dist_guia parameter; Bosters output; fase output; Cd_vertical output; Cd_lateral output; stop output; Vz input; distancia input; H input; t_ref output; Cd input

== matlab function simulation/Fligth stages/MATLAB Function ==
  data: u input; y output; v input
function y = fcn(u,v)

if u > v
    y = u;
else
    y = v;
end

end

== stateflow chart simulation/Translational motion/Chart ==
  state State1
    entry:
    out = [0;0;0];
  state State2
    during:
    out = in;
  (default) -> State1
  State1 -> State2 : [in(3) > 0]
  data: in input; out output

== matlab function simulation/Translational motion/Forças/Fases 0 - 3/Empuxo/Turbojato ==
  data: Empuxo_turbojato output; velocity input; T0 input; a input; P0 input; fase input; Consumo output; altura input
function [Empuxo_turbojato,Consumo]  = Motor_turbojato(velocity,T0,a,P0,fase,altura)

if fase < 4
    M0 = norm(velocity)/a;
    P0_P9 = 0.84;
    
    % INPUTS: 
            % Choices: M0 (Mach),T0 (Temperature),P0 (Pressure),Tt4 (power),
            % P0/P9.
            % Constants: pidmax (inlet), pib, pit, pin
            %            taut
            %            etac, etab, etam
            %            gammac, gammat, cpc, cpt
            %            hPR
            % Reference conditions: M0R, T0R, P0R, taurR, Tt4R, TdR, picR,
            % taucR
        
        pidmax = 0.95;
        pib = 0.95;
        pit = 0.655;
        pin = 0.9872;
        taut = 0.923;
        etac = 0.8879;
        etab = 0.99;
        gammac = 1.4;
        gammat = 1.3;
        cpc = 1004;
        cpt = 1239;
        hPR = 42.8e6;
        
        M0R = 0.03;
        T0R = 298.15;
        P0R = 101325;
        Tt4R = 914.95;
        picR = 2.25;
        mdotR = 0.55; %0.2;
         
         Rc = (gammac-1)*gammac*cpc;
         Rt = (gammat-1)*gammat*cpt;
         a0 = sqrt(gammac*Rc*T0);
         V0 = a0*M0;
         taur = 1 + (gammac-1)*0.5*(M0^2);
         pir = taur^(gammac/(gammac-1));
         
         Tt4 = Tt4R; % potência máxima
         
         if M0 <= 1 
             etar = 1;
         else
             etar = 1 - 0.075*(M0-1)^1.35;
         end
         
         pid = pidmax*etar;
         
         taulambda = cpt*Tt4/(cpc*T0);
         Tt2 = T0*taur;
         
         taurR = 1 + ((gammac-1)/2)*M0R^2;
         Tt2R = T0R*taurR;
         
         taucR = picR^((gammac-1)/gammac);
         tauc = 1 + (taucR-1)*(Tt4/Tt2)/(Tt4R/Tt2R);
         pic = (1+etac*(tauc-1))^(gammac/(gammac-1));
         
         f = (taulambda - taur*tauc)/(hPR*etab/(cpc*T0)-taulambda);
         taub = taulambda/(taur*tauc);
         
         Pt9_P9 = (P0_P9)*pir*pid*pic*pib*pit*pin;
         M9 = sqrt((2/(gammat-1))*((Pt9_P9)^((gammat-1)/gammat)-1));
         T9_T0 = (Tt4*taut/T0)/(Pt9_P9^((gammat-1)/gammat)); %%%%%%%%%%%
         V9_a0 = M9*sqrt(gammat*Rt*T9_T0/(gammac*Rc));
         pidR = pidmax;
         
         mdot = mdotR*P0*pir*pid*pic/(P0R*pir*pidR*picR)*sqrt(Tt4R/Tt4);
    
         F_mdot = a0*( (1+f)*V9_a0 - M0 + (1+f)*Rt*T9_T0*(1-P0_P9)/(Rc*gammac*V9_a0) );
         F = mdot*F_mdot;
         S = f/F_mdot;
         Consumo = S*mdot;
    
    Empuxo_turbojato = F;

    %%%%%% Empuxo
    Empuxo_turbojato = 282 - 0.0255*altura;
else
    Empuxo_turbojato = 0;
    Consumo = 0;
end
    
end

== matlab function simulation/Translational motion/Forças/Fases 0 - 3/Forças aerodinâmicas/MATLAB Function ==
  data: atitude input; u_perpendicular output; alfa output; vento_relativo input
function [u_perpendicular,alfa] = fcn(atitude,vento_relativo)

if norm(vento_relativo) == 0
    alfa = 0;
    u_perpendicular = [0;0;0];
else
    alfa = atan(norm(cross(atitude,-vento_relativo))/dot(atitude,-vento_relativo));
    u_perpendicular = - (- vento_relativo - norm(vento_relativo)*cos(alfa)*atitude);
    if norm(u_perpendicular) ~= 0
        u_perpendicular = u_perpendicular/norm(u_perpendicular);
    end
end

end

== matlab function simulation/Translational motion/Forças/Fases 0 - 3/Forças aerodinâmicas/MATLAB Function1 ==
  data: Velocidade input; Cd_total output; Velocidade_som input; rho input; mi input; Geometria parameter
function Cd_total  = Modelo_arrasto_Barrowman(Velocidade,Velocidade_som,rho,mi,Geometria)

% Correção para números de mach muito baixo ( < 0.015)
V = norm(Velocidade);
Mach = V/Velocidade_som;

if Mach < 0.015
    Mach = 0.015;
    V = Mach*Velocidade_som;
end
   
    
    L_total = Geometria(1);
    Rs = Geometria(2);
    N = Geometria(3);
    At = Geometria(4);
    A_ref = Geometria(5);
    Awb = Geometria(6);
    tr = Geometria(7);
    tau_L = Geometria(8);
    cr = Geometria(9);
    AR = Geometria(10);
    tau_C = Geometria(11);
    fn = Geometria(12);
    r = Geometria(13);
    s = Geometria(14);
    C = Geometria(15);
    
    %V = norm(Velocidade);


    % Constantes admensionais
    %Mach = V/Velocidade_som;                     % número de Mach
    Re = rho*L_total*V/mi;                       % número de Reynolds
    Re_cr = 51*(abs(Rs/L_total))^(-1.039);            % Reynolds crítico
    Re_sonic = rho*L_total*Velocidade_som/mi;

    % 1) Skin friction drag
    if Re < 5*(10^5)
        Cf = 0.0148;
    elseif Re > Re_cr
        Cf = 0.032*(Rs/L_total)^0.2;
    else
        Cf = 1/(1.5*log(abs(Re)) - 5.6)^2;
    end

    % 1.1) Compressible subsonic variation
    if Re < 5*(10^5)
        Cfc = Cf*(1 - 0.09*Mach^2);
    else
        Cfc = Cf*(1 - 0.12*Mach^2);
    end


    % 1.2) Total friction drag
    Cd_ft = 2*N*Cfc*(At/A_ref); % arrasto nas aletas

    fb = L_total/(2*r);
    Cd_fb = (1 + 0.5/fb)*Cfc*Awb/A_ref;  % arrasto no corpo do foguete

    Cd_friction = Cd_ft + Cd_fb;

    % cálculo do Cfc_sonic
    if Re_sonic < 5*(10^5)
        Cf = 1.328/sqrt(abs(Re_sonic));
    elseif Re_sonic > Re_cr
        Cf = 0.032*(Rs/L_total)^0.2;
    else
        Cf = 1/(3.46*log(Re_sonic) - 5.6)^2 - 1700/Re;
    end
    if Re_sonic < 5*(10^5)
        Cfc_sonic = Cf/(1 - 0.045)^(1/4);
    else
        Cfc_sonic = Cf/(1 - 0.15)^(0.58);
    end

    % 2) Pressure drag

    % 2.1) Tail pressure drag
    if Mach < 0.9
        delta_Cd = abs((1 - Mach^2))^-0.417 - 1;
    else
        delta_Cd = 1 - 1.5*(Mach - 0.9);
    end

    % leading edge drag
    Sr = tr/2;
    Cd_L = 2*N*(Sr/A_ref)*(cos(tau_L)^2)*delta_Cd; % (Sr - fin leading edge radius)

    % The trailing edge is zero because it's sharp.

    % thickness drag
    episilon = AR*(tr/cr)^(1/3);
    Cd_th1 = 1.15*((tr/cr)^(5/3))*(1.61 + episilon - sqrt(abs((episilon - 1.43)^2 + 0.578)));
    At1 = s*tr;
    k1 = (Cd_th1*A_ref/(Cfc_sonic*At1) - 4*(tr/cr)*cos(tau_C))/(120*((tr/cr)^4)*(cos(tau_C)^2));
    k = cos(tau_C)^2 + abs(( k1 ))^(2/3);

    Cd_th = N*Cfc*(At1/A_ref)*( 4*(tr/cr)*cos(tau_C) + 120*((tr/cr)^4)*(cos(tau_C)^2)/(abs(k - (Mach*cos(tau_C))^2 )^(3/2)) );


    % 2.2) Body pressure drag
    if C == 1 % cone
        a = 0.88;
        b = 0.7;
        c = 1.29;
    elseif C == 2 % ogive
        a = 0.88;
        b = 1;
        c = 2.22;
    else
        a = 0.88;
        b = 1;
        c = 2.22;
    end

    Cd_p = a/(fn + b)^c;
    k = 1 + abs( 6*Awb*Cfc_sonic/((fb^3)*A_ref/Cd_p) )^(5/3);
    Cd_p = 6*Awb*Cfc/abs(( (fb^3)*A_ref*(k - Mach^2) ))^0.6;

    % 2.3) Base drag
    Cd_b1 = 0.185; % hr = 0 + 1.15*hr/cr;     % a área da base é igual a área de referência
    k = 1 + (0.029^2)/(Cfc_sonic*(Awb/A_ref)*(Cd_b1^2));

    if Mach < 1
        Cd_b = 0.029/sqrt(abs((Cfc*(Awb/A_ref)*(k - Mach^2))));
    else
        Cd_b = Cd_b1*(0.88 + 0.12*exp(-3.58*(Mach - 1)));
    end
    
    Cd_pressure = Cd_L + Cd_th + Cd_p + Cd_b;

    Cd_total = real(Cd_friction + Cd_pressure);


if Mach == 0.015
    Cd_total = Cd_total*( 1.1 - 6.67*norm(Velocidade)/Velocidade_som );
end

end

== matlab function simulation/Translational motion/Vento relativo/Vento ==
  data: fase input; posicao input; vento_x output; tempo input; vento_y output; Vento_eixo_x parameter; Vento_eixo_y parameter
function [vento_x,vento_y] = fcn(fase,posicao,tempo, Vento_eixo_x, Vento_eixo_y)

%vento_x = Vento_eixo_x;

%vento_y = Vento_eixo_y;

% Está sendo considerado que o Vento_eixo_x foi medida a 2 m de altura.

if posicao(3) < 0
    h = 0;
else
    h = posicao(3);
end

if fase > 1
    vento_x = Vento_eixo_x*(h/2)^0.143;
    vento_y = - Vento_eixo_y*(h/2)^0.01;
else
    vento_x = 0;
    vento_y = 0;
end

end

== matlab function simulation/Fligth stages/MATLAB Function1 ==
  data: massa input; Cd input; g input; H output; rho input; A_ref parameter; v input; tempo input
function H = fcn(massa,Cd,g,rho,A_ref,v,tempo)
if tempo > 0
    k = 0.5*rho*Cd*A_ref;
    H = massa/(2*k)*log(abs((massa*g + k*v^2)/(massa*g)));
else
    H = 0;
end

end

== stateflow chart simulation/Angular motion/Atitude1/Chart ==
  state State2
    state Eixo_x
      during:
      if Px > 0
      theta = 0;
      else
      theta = 180;
      end
      if Pz == 0
      phi = 90;
      elseif Pz > 0
      phi = (180/pi)*atan( (sqrt(Px^2 + Py^2))/Pz );
      else
      phi = 180 +  (180/pi)*atan( (sqrt(Px^2 + Py^2))/Pz );
      end
    state State1
      during:
      if (Px > 0) && (Py > 0)
      theta = (180/pi)*atan(Py/Px);
      elseif (Px < 0) && (Py > 0)
      theta = 180 -  (180/pi)*atan(-Py/Px);
      elseif (Px < 0) && (Py < 0)
      theta = 270 -  (180/pi)*atan(Py/Px);
      elseif (Px > 0) && (Py < 0)
      theta = 360 -  (180/pi)*atan(-Py/Px);
      end
      if Pz == 0
      phi = 90;
      elseif Pz > 0
      phi = (180/pi)*atan( (sqrt(Px^2 + Py^2))/Pz );
      else
      phi = 180 +  (180/pi)*atan( (sqrt(Px^2 + Py^2))/Pz );
      end
    state Origem
      entry:
      phi = 0;
      theta = 0;
    state Eixo_y
      during:
      if Py > 0
      theta = 90;
      else
      theta = 270;
      end
      if Pz == 0
      phi = 90;
      elseif Pz > 0
      phi = (180/pi)*atan( (sqrt(Px^2 + Py^2))/Pz );
      else
      phi = 180 + (180/pi)*atan( (sqrt(Px^2 + Py^2))/Pz );
      end
    Eixo_x -> State1 [order 1] : [(Px ~= 0)&&(Py ~= 0)]
    Origem -> Eixo_x [order 2] : [(Px~= 0)&&(Py == 0)]
    State1 -> Eixo_x [order 1] : [(Px~= 0)&&(Py == 0)]
    Eixo_x -> Origem [order 3] : [(Px == 0)&&(Py == 0)]
    Eixo_y -> Eixo_x [order 2] : [(Px~= 0)&&(Py == 0)]
    Eixo_x -> Eixo_y [order 2] : [(Py ~= 0)&&(Px == 0)]
    State1 -> Origem [order 3] : [(Px == 0)&&(Py == 0)]
    (default) -> Origem
    Origem -> State1 [order 3] : [(Px ~= 0)&&(Py ~= 0)]
    Origem -> Eixo_y [order 1] : [(Py ~= 0)&&(Px == 0)]
    Eixo_y -> Origem [order 3] : [(Px == 0)&&(Py == 0)]
    Eixo_y -> State1 [order 1] : [(Px ~= 0)&&(Py ~= 0)]
    State1 -> Eixo_y [order 2] : [(Py ~= 0)&&(Px == 0)]
  state State3
    entry:
    phi = 0;
    theta = 0;
  (default) -> State2
  State2 -> State3 : [fase >= 5]
  data: Px input; Py input; Pz input; phi output; theta output; fase input

== matlab function simulation/Angular motion/Atitude1/MATLAB Function ==
  data: fase input; v input; alfa output; a input
function alfa = fcn(fase,v,a)
if (norm(v) ~= 0) && (fase < 5) && (fase > 2)
    alfa = abs(atand(norm(cross(v,a))/dot(v,a)));
else
    alfa = 0;
end
end

== matlab function simulation/Angular motion/MATLAB Function ==
  data: s input; y output; v input; r input
function y = fcn(s,v,r)

y = s*s*r - dot(v,v)*r + 2*dot(v,r)*v + 2*s*cross(v,r);

end

== stateflow chart simulation/Angular motion/Quaternion rotação1/Chart ==
  state state1
    entry:
    y = [a0;a1;a2;a3];
    d = y;
  state state2
    during:
    vec_u = [a1;a2;a3];
    vec_c = [c(2);c(3);c(4)];
    escalar = a0*c(1) - dot(vec_u,vec_c);
    vetor = a0*vec_c + c(1)*vec_u + cross(vec_u,vec_c);
    y = [escalar;vetor];
    d = y;
  (default) -> state1
  state1 -> state2 : [time > 0]
  data: time input; a0 input; a1 input; a2 input; a3 input; c input; y output; d output; vec_c local; vec_u local; escalar local; vetor local
